simulink model "M1DCS_2_rust"  (R2022b)
settings: Solver=FixedStepDiscrete  StartTime=0.0  StopTime=5  FixedStep=deltaT  RelTol=1e-3
InitFcn:
  | %
  | % Initialization callback function
  | %
  | 
  | try
  |    % fprintf('\n Simulink control model!\n');
  | 
  |    % Get Simulink model directory
  |    [filepath,name,ext] = fileparts(which(bdroot));
  | 
  |    if ~strcmp(filepath,pwd)
  |       fprintf('\n Changing current directory to \n %s \n',filepath);
  |       cd(filepath);
  |    end
  | 
  | catch
  |    warning('Running the InitFcn from puSimulate script');
  | end
values from neighbouring files (symbols this model uses):
  CS_Kbal = [0.000534994973474 0.00340191071412 -9.47788829769e-05 0.00343343348513 -0.000647828526781 -0.000556821142243 -0.000534821819969 -0.00340176071448 9.48233962239e-05 -0.00343325428788 0.000647837590074 0.000556848416436 ... (1836 elements, 306x6)]    [SupportActuatorArrayConfig.mat]
  CS_ofl_SSdtC = ofl_SSdtC    [load_M1DCS_data.m]
  H_p_cyl_DT = c2d(H_p_cyl, T_ofl, 'foh')    [load_M1DCS_data.m]
  HPdyn = c2d(feedback(tf([kpp_, kpi_],[1 0])*Hv_*Pp,1), T_ofl,'foh')    [load_M1DCS_data.m]
  m1_HPk = mean(HPstiffvec)    [load_M1DCS_data.m]
  M_HP_OA = M_HP_OA + (1/6)*M_HP_seg{i_}    [load_M1DCS_data.m]
  OA_Kbal = [0.0131193522784 0 0.000573456323239 0.0120863820226 0 -0.000305081290389 0.0117152923831 0 0.000463979607413 0.0115338103781 0 -0.00185896787401 ... (2010 elements, 335x6)]    [SupportActuatorArrayConfig.mat]
  OA_ofl_SSdtC = ofl_SSdtC    [load_M1DCS_data.m]
  T_ofl = 0.01    [load_M1DCS_data.m]
undefined symbols (not defined in the file or in its folder): m1sys, M_HP_CS, S1_M1RBM2HP, S2_M1RBM2HP, S3_M1RBM2HP, S4_M1RBM2HP, S5_M1RBM2HP, S6_M1RBM2HP, S7_M1RBM2HP
libraries: ims_block_library x2
settings Model: SimulationMode=accelerator  Creator=RRomano  LastModifiedBy=rromano
settings SolverCC: AlgebraicLoopSolver=TrustRegion
settings DataIOCC: SaveOutput=off  SignalLogging=off  DSMLogging=off  SaveTime=off  ReturnWorkspaceOutputs=off
settings OptimizationCC: DefaultParameterBehavior=Inlined  GainParamInheritBuiltInType=on  UseFloatMulNetSlope=on  UseSpecifiedMinMax=on  InlineInvariantSignals=on  StrengthReduction=on  PassReuseOutputArgsAs=Individual arguments  ZeroExternalMemoryAtStartup=off  ZeroInternalMemoryAtStartup=off  NoFixptDivByZeroProtection=on  EfficientFloat2IntCast=on  LifeSpan=1000  SimCompilerOptimization=on  AccelVerboseBuild=on  OptimizeBlockOrder=speed  OptimizationPriority=Speed  OptimizationCustomize=off  MultiThreadedLoops=on  EfficientTunableParamExpr=on
settings DebuggingCC: InheritedTsInSrcMsg=none  MultiTaskRateTransMsg=warning  ParameterTunabilityLossMsg=error  UnconnectedInputMsg=warning  UnconnectedOutputMsg=warning  UnconnectedLineMsg=warning  SFUnexpectedBacktrackingDiag=warning  SFNoUnconditionalDefaultTransitionDiag=warning  SFExecutionAtInitializationDiag=none  SFMachineParentedDataDiag=warning  ArithmeticOperatorsInVariantConditions=warning
settings HardwareCC: ProdBitPerLong=64  ProdLongLongMode=on  ProdHWDeviceType=Intel->x86-64 (Linux 64)  TargetBitPerLong=64  TargetBitPerPointer=64  TargetBitPerSizeT=64  TargetBitPerPtrDiffT=64  TargetLongLongMode=on  TargetIntDivRoundTo=Zero  TargetEndianess=LittleEndian  TargetWordSize=64  TargetHWDeviceType=MATLAB Host  ProdEqTarget=off
settings ModelReferenceCC: EnableRefExpFcnMdlSchedulingChecks=on
settings SFSimCC: SimUseLocalCustomCode=off  MATLABDynamicMemAlloc=off  CustomCodeUndefinedFunction=UseInterfaceOnly
settings RTWCC: Description=Embedded Coder  SystemTargetFile=ert.tlc  GenCodeOnly=on  GenerateMakefile=off  TemplateMakefile=ert_default_tmf  GenerateReport=on  BuildConfiguration=Faster Runs  RTWCompilerOptimization=on  CheckMdlBeforeBuild=Warning  DLArmComputeVersion=19.05
settings CodeAppCC: ForceParamTrailComments=on  IgnoreCustomStorageClasses=off  OperatorAnnotations=on  SimulinkDataObjDesc=on  SFDataObjDesc=on  InsertBlockDesc=on
settings ERTTargetCC: TargetLangStandard=C99 (ISO)  GenerateSampleERTMain=on  CombineSignalStateStructs=on  SuppressErrorStatus=on  CodeInterfacePackaging=Reusable function  SupportNonFinite=off  SupportComplex=off  InlinedParameterPlacement=NonHierarchical  RootIOFormat=Structure reference  ERTCustomFileTemplate=example_file_process.tlc
settings ConfigComp: CovMetricSettings=dw  CovSaveCumulativeToWorkspaceVar=on  CovSaveSingleToWorkspaceVar=on  CovExternalEMLEnable=off

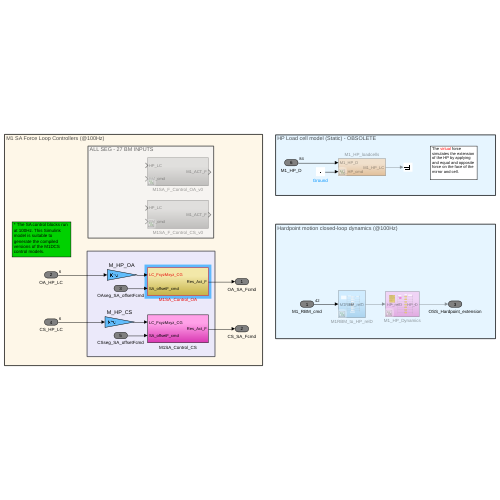
[thumbnail: Simulink's stored preview of the top-level diagram]
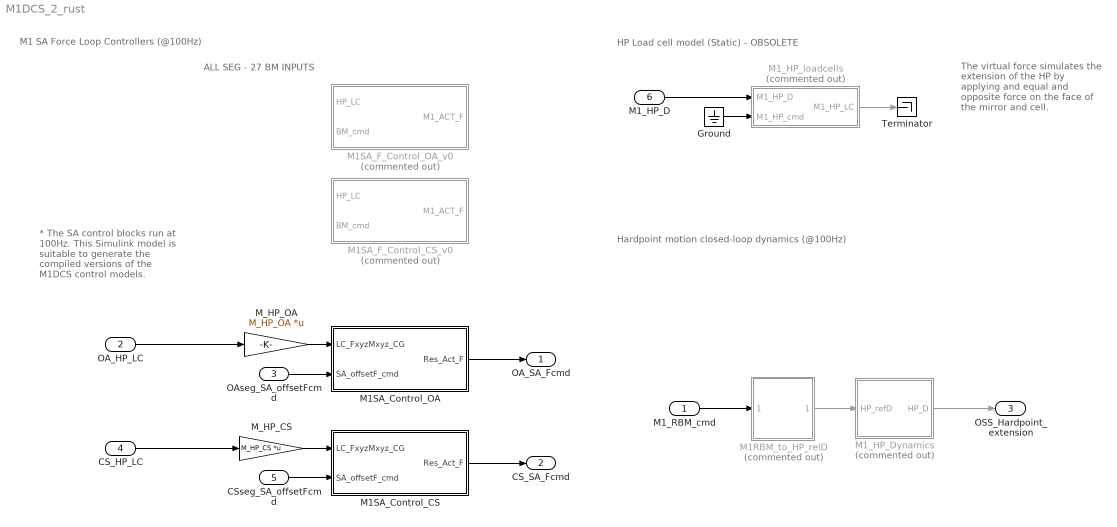
== system M1DCS_2_rust ==
  note: HP Load cell model (Static) - OBSOLETE
  note: Hardpoint motion closed-loop dynamics (@100Hz)
  note: ALL SEG - 27 BM INPUTS
  note: * The SA control blocks run at 100Hz. This Simulink model is suitable to generate the compiled versions of the M1DCS control models.
  note: M1 SA Force Loop Controllers (@100Hz)
  note: The virtual force simulates the extension of the HP by applying and equal and opposite force on the face of the mirror and cell.
  M1_RBM_cmd : Inport  PortDimensions=42
  OA_HP_LC : Inport  Port=2  PortDimensions=size(M_HP_OA,2)  SampleTime=T_ofl
  OAseg_SA_offsetFcmd : Inport  Port=3  SampleTime=T_ofl
  CS_HP_LC : Inport  Port=4  PortDimensions=size(M_HP_CS,2)  SampleTime=T_ofl
  CSseg_SA_offsetFcmd : Inport  Port=5  SampleTime=T_ofl
  M1_HP_D : Inport  Port=6  PortDimensions=84
  Ground : Ground
  M1RBM_to_HP_relD : Subsystem  Commented=on
  M1SA_Control_CS : Subsystem
  M1SA_Control_OA : Subsystem
  M1SA_F_Control_CS_v0 : Subsystem  Commented=on
  M1SA_F_Control_OA_v0 : Subsystem  Commented=on
  M1_HP_Dynamics : Subsystem  Commented=on
  M1_HP_loadcells : Subsystem  Commented=on
  M_HP_CS : Gain  Gain=M_HP_CS  Multiplication=Matrix(K*u)
  M_HP_OA : Gain  Gain=M_HP_OA  Multiplication=Matrix(K*u)
  Terminator : Terminator
  OA_SA_Fcmd : Outport  SampleTime=T_ofl  VectorParamsAs1DForOutWhenUnconnected=off
  CS_SA_Fcmd : Outport  Port=2  SampleTime=T_ofl  VectorParamsAs1DForOutWhenUnconnected=off
  OSS_Hardpoint_extension : Outport  Port=3  VectorParamsAs1DForOutWhenUnconnected=off
  wires:
  M1_RBM_cmd/1 -> M1RBM_to_HP_relD/1(M1RBM)
  M1SA_Control_CS/1(Res_Act_F) -> CS_SA_Fcmd/1
  CSseg_SA_offsetFcmd/1 -> M1SA_Control_CS/2(SA_offsetF_cmd)
  CS_HP_LC/1 -> M_HP_CS/1
  M1SA_Control_OA/1(Res_Act_F) -> OA_SA_Fcmd/1
  OA_HP_LC/1 -> M_HP_OA/1
  OAseg_SA_offsetFcmd/1 -> M1SA_Control_OA/2(SA_offsetF_cmd)
  M_HP_OA/1 -> M1SA_Control_OA/1(LC_FxyzMxyz_CG)
  M_HP_CS/1 -> M1SA_Control_CS/1(LC_FxyzMxyz_CG)
  M1_HP_Dynamics/1(HP_D) -> OSS_Hardpoint_extension/1
  M1RBM_to_HP_relD/1(HP_relD) -> M1_HP_Dynamics/1(HP_refD)
  M1_HP_loadcells/1(M1_HP_LC) -> Terminator/1
  M1_HP_D/1 -> M1_HP_loadcells/1(M1_HP_D)
  Ground/1 -> M1_HP_loadcells/2(M1_HP_cmd)

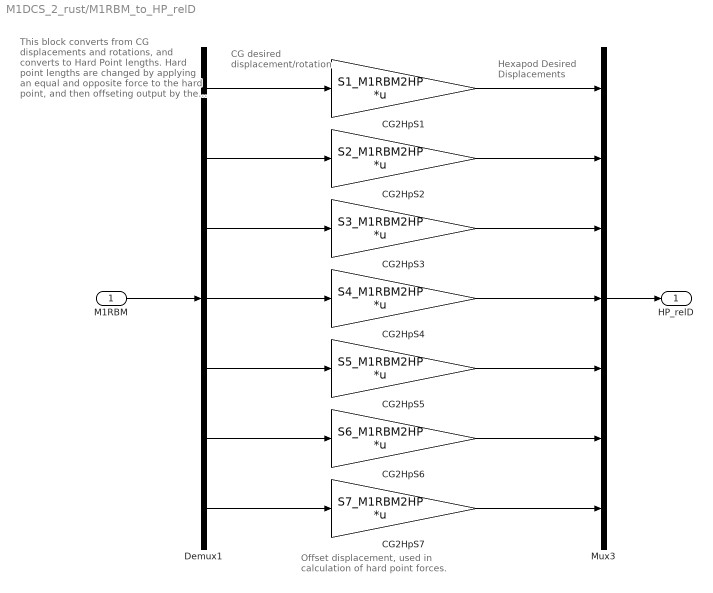
== system M1DCS_2_rust/M1RBM_to_HP_relD ==
  note: CG desired
      | displacement/rotation
  note: This block converts from CG displacements and rotations,
      | and converts to Hard Point lengths.  Hard point lengths are
      | changed by applying an equal and opposite force to the hard
      | point, and then offseting output by the commanded change
      | in position.
  note: Hexapod Desired
      | Displacements
  note: Offset displacement, used in calculation of hard point forces.
  M1RBM : Inport
  CG2HpS1 : Gain  Gain=S1_M1RBM2HP  Multiplication=Matrix(K*u)
  CG2HpS2 : Gain  Gain=S2_M1RBM2HP  Multiplication=Matrix(K*u)
  CG2HpS3 : Gain  Gain=S3_M1RBM2HP  Multiplication=Matrix(K*u)
  CG2HpS4 : Gain  Gain=S4_M1RBM2HP  Multiplication=Matrix(K*u)
  CG2HpS5 : Gain  Gain=S5_M1RBM2HP  Multiplication=Matrix(K*u)
  CG2HpS6 : Gain  Gain=S6_M1RBM2HP  Multiplication=Matrix(K*u)
  CG2HpS7 : Gain  Gain=S7_M1RBM2HP  Multiplication=Matrix(K*u)
  Demux1 : Demux  Outputs=6*ones(7,1)
  Mux3 : Mux  Inputs=6*ones(7,1)
  HP_relD : Outport  VectorParamsAs1DForOutWhenUnconnected=off
  wires:
  Mux3/1 -> HP_relD/1
  Demux1/2 -> CG2HpS2/1
  Demux1/3 -> CG2HpS3/1
  Demux1/4 -> CG2HpS4/1
  Demux1/5 -> CG2HpS5/1
  Demux1/6 -> CG2HpS6/1
  Demux1/1 -> CG2HpS1/1
  Demux1/7 -> CG2HpS7/1
  CG2HpS1/1 -> Mux3/1
  M1RBM/1 -> Demux1/1
  CG2HpS2/1 -> Mux3/2
  CG2HpS3/1 -> Mux3/3
  CG2HpS4/1 -> Mux3/4
  CG2HpS5/1 -> Mux3/5
  CG2HpS6/1 -> Mux3/6
  CG2HpS7/1 -> Mux3/7

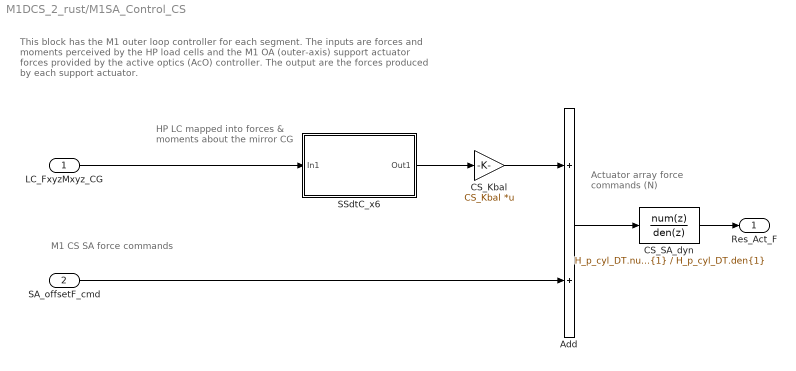
== system M1DCS_2_rust/M1SA_Control_CS ==
  note: This block has the M1 outer loop controller for each segment. The inputs are forces and moments perceived by the HP load cells and the M1 OA (outer-axis) support actuator forces provided by the active optics (AcO) controller. The output are the forces produced by each support actuator.
  note: Actuator array
      | force commands (N)
  note: M1 CS SA
      | force commands
  note: HP LC mapped into forces & moments about the mirror CG
  LC_FxyzMxyz_CG : Inport  PortDimensions=size(M_HP_CS,1)  SampleTime=T_ofl
  SA_offsetF_cmd : Inport  Port=2  PortDimensions=size(CS_Kbal,1)  SampleTime=T_ofl
  Add : Sum
  CS_Kbal : Gain  Gain=CS_Kbal  Multiplication=Matrix(K*u)
  CS_SA_dyn : DiscreteTransferFcn  Numerator=H_p_cyl_DT.num{1}  Denominator=H_p_cyl_DT.den{1}  SampleTime=T_ofl  a0EqualsOne=on
  SSdtC_x6 : Subsystem
  Res_Act_F : Outport  VectorParamsAs1DForOutWhenUnconnected=off
  wires:
  Add/1 -> CS_SA_dyn/1
  SA_offsetF_cmd/1 -> Add/2
  LC_FxyzMxyz_CG/1 -> SSdtC_x6/1(In1)
  SSdtC_x6/1(Out1) -> CS_Kbal/1
  CS_Kbal/1 -> Add/1
  CS_SA_dyn/1 -> Res_Act_F/1

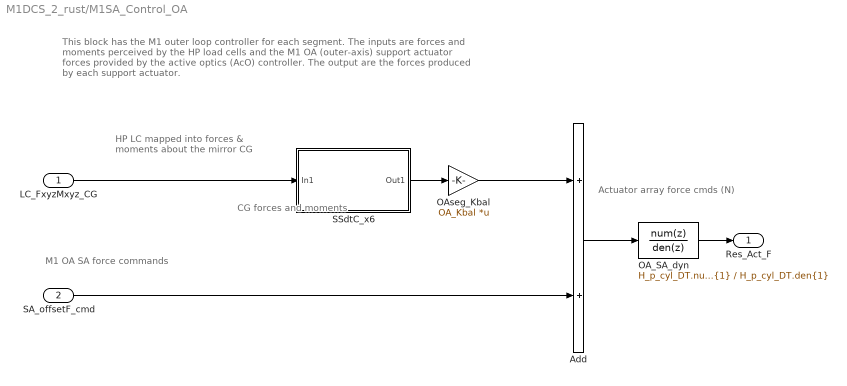
== system M1DCS_2_rust/M1SA_Control_OA ==
  note: M1 OA SA force
      | commands
  note: This block has the M1 outer loop controller for each segment. The inputs are forces and moments perceived by the HP load cells and the M1 OA (outer-axis) support actuator forces provided by the active optics (AcO) controller. The output are the forces produced by each support actuator.
  note: CG forces
      | and moments
  note: Actuator array
      | force cmds (N)
  note: HP LC mapped into forces & moments about the mirror CG
  LC_FxyzMxyz_CG : Inport  PortDimensions=size(M_HP_OA,1)  SampleTime=T_ofl
  SA_offsetF_cmd : Inport  Port=2  PortDimensions=size(OA_Kbal,1)  SampleTime=T_ofl
  Add : Sum
  OA_SA_dyn : DiscreteTransferFcn  Numerator=H_p_cyl_DT.num{1}  Denominator=H_p_cyl_DT.den{1}  SampleTime=T_ofl  a0EqualsOne=on
  OAseg_Kbal : Gain  Gain=OA_Kbal  Multiplication=Matrix(K*u)
  SSdtC_x6 : Subsystem
  Res_Act_F : Outport  VectorParamsAs1DForOutWhenUnconnected=off
  wires:
  SA_offsetF_cmd/1 -> Add/2
  OAseg_Kbal/1 -> Add/1
  LC_FxyzMxyz_CG/1 -> SSdtC_x6/1(In1)
  SSdtC_x6/1(Out1) -> OAseg_Kbal/1
  OA_SA_dyn/1 -> Res_Act_F/1
  Add/1 -> OA_SA_dyn/1

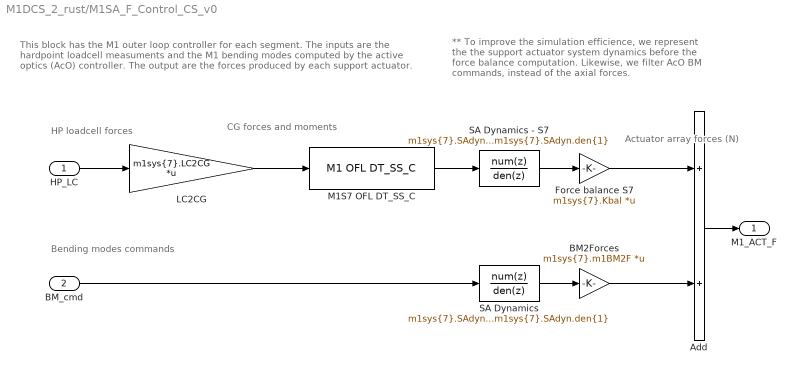
== system M1DCS_2_rust/M1SA_F_Control_CS_v0 ==
  note: This block has the M1 outer loop controller for each segment. The inputs are the hardpoint loadcell measuments and the M1 bending modes computed by the active optics (AcO) controller. The output are the forces produced by each support actuator.
  note: Actuator array
      | forces (N)
  note: HP loadcell
      | forces
  note: ** To improve the simulation efficience, we represent the the support actuator system dynamics before the force balance computation. Likewise, we filter AcO BM commands, instead of the axial forces.
  note: Bending modes
      | commands
  note: CG forces
      | and moments
  HP_LC : Inport  PortDimensions=size(m1sys{7}.LC2CG,1)  SampleTime=m1sys{7}.ofl.SSdtC{1}.Ts
  BM_cmd : Inport  Port=2  PortDimensions=n_bm  SampleTime=m1sys{7}.ofl.SSdtC{1}.Ts
  Add : Sum
  BM2Forces : Gain  Gain=m1sys{7}.m1BM2F  Multiplication=Matrix(K*u)
  Force balance S7 : Gain  Gain=m1sys{7}.Kbal  Multiplication=Matrix(K*u)
  LC2CG : Gain  Gain=m1sys{7}.LC2CG  Multiplication=Matrix(K*u)
  M1S7 OFL DT_SS_C : ims_block_library/M1 OFL DT_SS_C  dt_SS_struct=m1sys{7}.ofl.SSdtC
  SA Dynamics : DiscreteTransferFcn  Numerator=m1sys{7}.SAdyn.num{1}  Denominator=m1sys{7}.SAdyn.den{1}  SampleTime=m1sys{7}.ofl.SSdtC{1}.Ts  a0EqualsOne=on
  SA Dynamics - S7 : DiscreteTransferFcn  Numerator=m1sys{7}.SAdyn.num{1}  Denominator=m1sys{7}.SAdyn.den{1}  SampleTime=m1sys{7}.ofl.SSdtC{1}.Ts  a0EqualsOne=on
  M1_ACT_F : Outport  VectorParamsAs1DForOutWhenUnconnected=off
  wires:
  Force balance S7/1 -> Add/1
  Add/1 -> M1_ACT_F/1
  HP_LC/1 -> LC2CG/1
  SA Dynamics - S7/1 -> Force balance S7/1
  BM2Forces/1 -> Add/2
  M1S7 OFL DT_SS_C/1 -> SA Dynamics - S7/1
  LC2CG/1 -> M1S7 OFL DT_SS_C/1
  BM_cmd/1 -> SA Dynamics/1
  SA Dynamics/1 -> BM2Forces/1

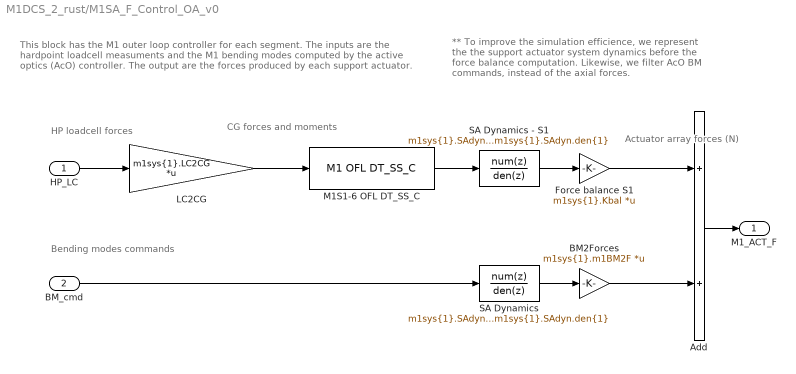
== system M1DCS_2_rust/M1SA_F_Control_OA_v0 ==
  note: ** To improve the simulation efficience, we represent the the support actuator system dynamics before the force balance computation. Likewise, we filter AcO BM commands, instead of the axial forces.
  note: Bending modes
      | commands
  note: This block has the M1 outer loop controller for each segment. The inputs are the hardpoint loadcell measuments and the M1 bending modes computed by the active optics (AcO) controller. The output are the forces produced by each support actuator.
  note: CG forces
      | and moments
  note: Actuator array
      | forces (N)
  note: HP loadcell
      | forces
  HP_LC : Inport  PortDimensions=size(m1sys{1}.LC2CG,1)  SampleTime=m1sys{1}.ofl.SSdtC{1}.Ts
  BM_cmd : Inport  Port=2  PortDimensions=n_bm  SampleTime=m1sys{1}.ofl.SSdtC{1}.Ts
  Add : Sum
  BM2Forces : Gain  Gain=m1sys{1}.m1BM2F  Multiplication=Matrix(K*u)
  Force balance S1 : Gain  Gain=m1sys{1}.Kbal  Multiplication=Matrix(K*u)
  LC2CG : Gain  Gain=m1sys{1}.LC2CG  Multiplication=Matrix(K*u)
  M1S1-6 OFL DT_SS_C : ims_block_library/M1 OFL DT_SS_C  dt_SS_struct=m1sys{1}.ofl.SSdtC
  SA Dynamics : DiscreteTransferFcn  Numerator=m1sys{1}.SAdyn.num{1}  Denominator=m1sys{1}.SAdyn.den{1}  SampleTime=m1sys{1}.ofl.SSdtC{1}.Ts  a0EqualsOne=on
  SA Dynamics - S1 : DiscreteTransferFcn  Numerator=m1sys{1}.SAdyn.num{1}  Denominator=m1sys{1}.SAdyn.den{1}  SampleTime=m1sys{1}.ofl.SSdtC{1}.Ts  a0EqualsOne=on
  M1_ACT_F : Outport  VectorParamsAs1DForOutWhenUnconnected=off
  wires:
  Force balance S1/1 -> Add/1
  M1S1-6 OFL DT_SS_C/1 -> SA Dynamics - S1/1
  HP_LC/1 -> LC2CG/1
  SA Dynamics - S1/1 -> Force balance S1/1
  BM_cmd/1 -> SA Dynamics/1
  LC2CG/1 -> M1S1-6 OFL DT_SS_C/1
  Add/1 -> M1_ACT_F/1
  SA Dynamics/1 -> BM2Forces/1
  BM2Forces/1 -> Add/2

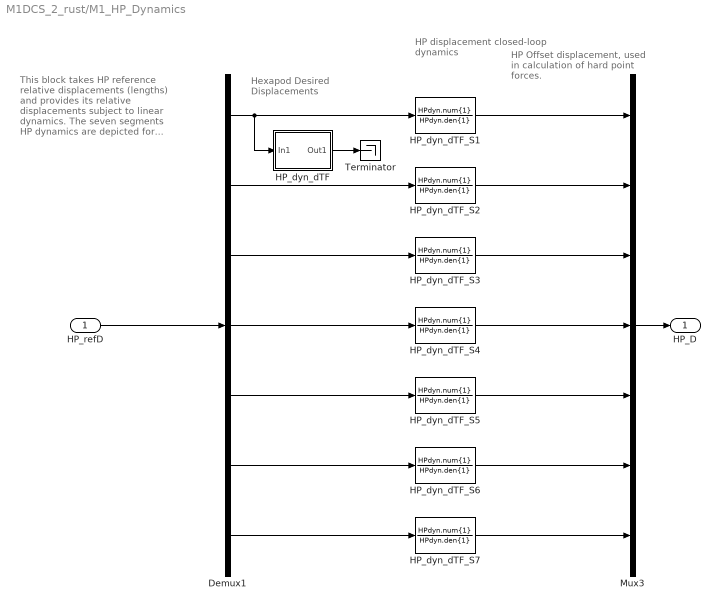
== system M1DCS_2_rust/M1_HP_Dynamics ==
  note: This block takes HP reference relative displacements (lengths) and provides its relative displacements subject to linear dynamics. The seven segments HP dynamics are depicted for illustration. One is supposed to build the single segmen dynamcs ( magenta block HP_dyn_dTF ). Then, the code is cloned for the multiple segments.
  note: Hexapod Desired
      | Displacements
  note: HP Offset displacement, used in calculation of hard point forces.
  note: HP displacement closed-loop dynamics
  HP_refD : Inport
  Demux1 : Demux  Outputs=6*ones(7,1)
  HP_dyn_dTF : Subsystem
  HP_dyn_dTF_S{1..7} (7 alike) : DiscreteTransferFcn  Numerator=HPdyn.num{1}  Denominator=HPdyn.den{1}  SampleTime=HPdyn.Ts  a0EqualsOne=on
  Mux3 : Mux  Inputs=6*ones(7,1)
  Terminator : Terminator
  HP_D : Outport  VectorParamsAs1DForOutWhenUnconnected=off
  wires:
  Mux3/1 -> HP_D/1
  Demux1/1 -> HP_dyn_dTF/1(In1), HP_dyn_dTF_S1/1
  HP_refD/1 -> Demux1/1
  Demux1/2 -> HP_dyn_dTF_S2/1
  Demux1/3 -> HP_dyn_dTF_S3/1
  Demux1/4 -> HP_dyn_dTF_S4/1
  Demux1/5 -> HP_dyn_dTF_S5/1
  Demux1/6 -> HP_dyn_dTF_S6/1
  Demux1/7 -> HP_dyn_dTF_S7/1
  HP_dyn_dTF_S1/1 -> Mux3/1
  HP_dyn_dTF_S2/1 -> Mux3/2
  HP_dyn_dTF_S3/1 -> Mux3/3
  HP_dyn_dTF_S4/1 -> Mux3/4
  HP_dyn_dTF_S5/1 -> Mux3/5
  HP_dyn_dTF_S6/1 -> Mux3/6
  HP_dyn_dTF_S7/1 -> Mux3/7
  HP_dyn_dTF/1(Out1) -> Terminator/1

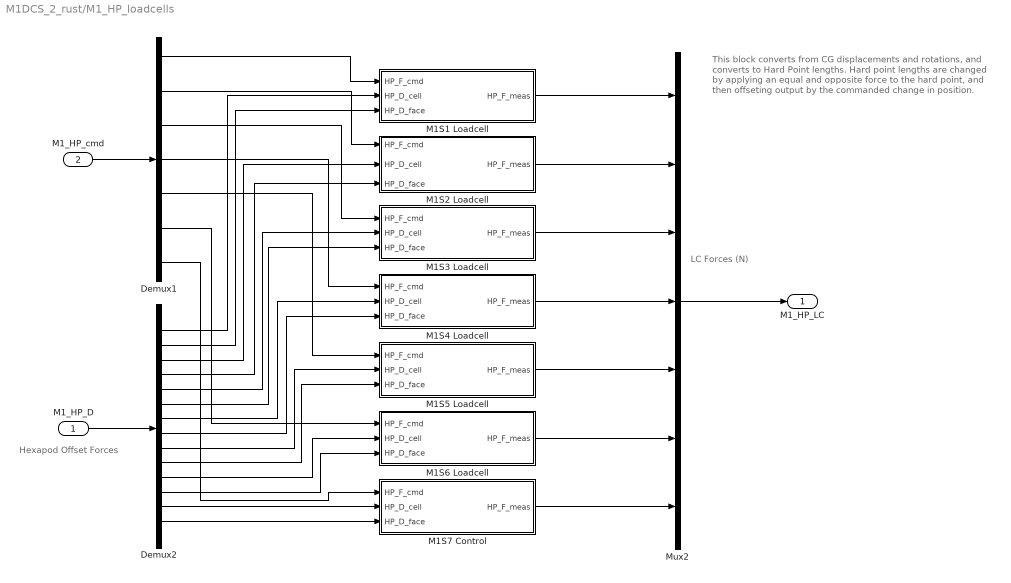
== system M1DCS_2_rust/M1_HP_loadcells ==
  note: This block converts from CG displacements and rotations,
      | and converts to Hard Point lengths.  Hard point lengths are
      | changed by applying an equal and opposite force to the hard
      | point, and then offseting output by the commanded change
      | in position.
  note: Hexapod Offset Forces
  note: LC Forces (N)
  M1_HP_D : Inport
  M1_HP_cmd : Inport  Port=2
  Demux1 : Demux  Outputs=6*ones(7,1)
  Demux2 : Demux  Outputs=6*ones(14,1);%6*ones(7,1)
  M1S1 Loadcell : Subsystem
  M1S2 Loadcell : Subsystem
  M1S3 Loadcell : Subsystem
  M1S4 Loadcell : Subsystem
  M1S5 Loadcell : Subsystem
  M1S6 Loadcell : Subsystem
  M1S7 Control : Subsystem
  Mux2 : Mux  Inputs=7
  M1_HP_LC : Outport  VectorParamsAs1DForOutWhenUnconnected=off
  wires:
  Demux2/9 -> M1S5 Loadcell/2(HP_D_cell)
  Demux2/3 -> M1S2 Loadcell/2(HP_D_cell)
  Demux2/5 -> M1S3 Loadcell/2(HP_D_cell)
  Demux2/13 -> M1S7 Control/2(HP_D_cell)
  Demux2/11 -> M1S6 Loadcell/2(HP_D_cell)
  Demux2/4 -> M1S2 Loadcell/3(HP_D_face)
  Demux2/6 -> M1S3 Loadcell/3(HP_D_face)
  Demux2/10 -> M1S5 Loadcell/3(HP_D_face)
  Demux2/12 -> M1S6 Loadcell/3(HP_D_face)
  Demux2/14 -> M1S7 Control/3(HP_D_face)
  M1_HP_D/1 -> Demux2/1
  M1S1 Loadcell/1(HP_F_meas) -> Mux2/1
  M1S2 Loadcell/1(HP_F_meas) -> Mux2/2
  M1S3 Loadcell/1(HP_F_meas) -> Mux2/3
  M1S5 Loadcell/1(HP_F_meas) -> Mux2/5
  M1S6 Loadcell/1(HP_F_meas) -> Mux2/6
  M1S7 Control/1(HP_F_meas) -> Mux2/7
  Demux2/2 -> M1S1 Loadcell/3(HP_D_face)
  Demux2/1 -> M1S1 Loadcell/2(HP_D_cell)
  M1S4 Loadcell/1(HP_F_meas) -> Mux2/4
  Demux2/7 -> M1S4 Loadcell/2(HP_D_cell)
  Demux2/8 -> M1S4 Loadcell/3(HP_D_face)
  M1_HP_cmd/1 -> Demux1/1
  Demux1/1 -> M1S1 Loadcell/1(HP_F_cmd)
  Demux1/2 -> M1S2 Loadcell/1(HP_F_cmd)
  Demux1/3 -> M1S3 Loadcell/1(HP_F_cmd)
  Demux1/4 -> M1S4 Loadcell/1(HP_F_cmd)
  Demux1/5 -> M1S5 Loadcell/1(HP_F_cmd)
  Demux1/6 -> M1S6 Loadcell/1(HP_F_cmd)
  Demux1/7 -> M1S7 Control/1(HP_F_cmd)
  Mux2/1 -> M1_HP_LC/1

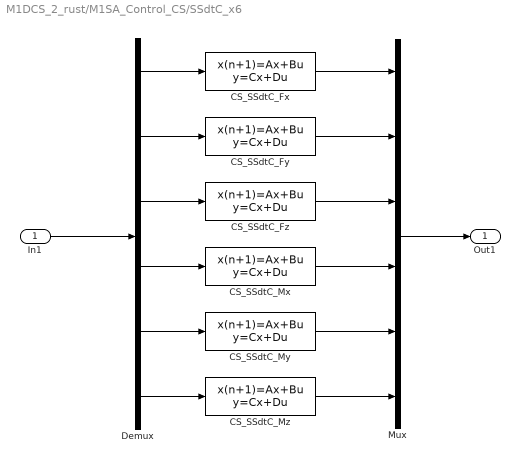
== system M1DCS_2_rust/M1SA_Control_CS/SSdtC_x6 ==
  In1 : Inport
  CS_SSdtC_Fx : DiscreteStateSpace  A=CS_ofl_SSdtC.A  B=CS_ofl_SSdtC.B  C=CS_ofl_SSdtC.C  D=CS_ofl_SSdtC.D  SampleTime=CS_ofl_SSdtC.Ts
  CS_SSdtC_Fy : DiscreteStateSpace  A=CS_ofl_SSdtC.A  B=CS_ofl_SSdtC.B  C=CS_ofl_SSdtC.C  D=CS_ofl_SSdtC.D  SampleTime=CS_ofl_SSdtC.Ts
  CS_SSdtC_Fz : DiscreteStateSpace  A=CS_ofl_SSdtC.A  B=CS_ofl_SSdtC.B  C=CS_ofl_SSdtC.C  D=CS_ofl_SSdtC.D  SampleTime=CS_ofl_SSdtC.Ts
  CS_SSdtC_Mx : DiscreteStateSpace  A=CS_ofl_SSdtC.A  B=CS_ofl_SSdtC.B  C=CS_ofl_SSdtC.C  D=CS_ofl_SSdtC.D  SampleTime=CS_ofl_SSdtC.Ts
  CS_SSdtC_My : DiscreteStateSpace  A=CS_ofl_SSdtC.A  B=CS_ofl_SSdtC.B  C=CS_ofl_SSdtC.C  D=CS_ofl_SSdtC.D  SampleTime=CS_ofl_SSdtC.Ts
  CS_SSdtC_Mz : DiscreteStateSpace  A=CS_ofl_SSdtC.A  B=CS_ofl_SSdtC.B  C=CS_ofl_SSdtC.C  D=CS_ofl_SSdtC.D  SampleTime=CS_ofl_SSdtC.Ts
  Demux : Demux  Outputs=6
  Mux : Mux  Inputs=6
  Out1 : Outport
  wires:
  In1/1 -> Demux/1
  Demux/1 -> CS_SSdtC_Fx/1
  CS_SSdtC_Fx/1 -> Mux/1
  Mux/1 -> Out1/1
  Demux/2 -> CS_SSdtC_Fy/1
  CS_SSdtC_Fy/1 -> Mux/2
  Demux/3 -> CS_SSdtC_Fz/1
  CS_SSdtC_Fz/1 -> Mux/3
  Demux/4 -> CS_SSdtC_Mx/1
  CS_SSdtC_Mx/1 -> Mux/4
  Demux/5 -> CS_SSdtC_My/1
  CS_SSdtC_My/1 -> Mux/5
  Demux/6 -> CS_SSdtC_Mz/1
  CS_SSdtC_Mz/1 -> Mux/6

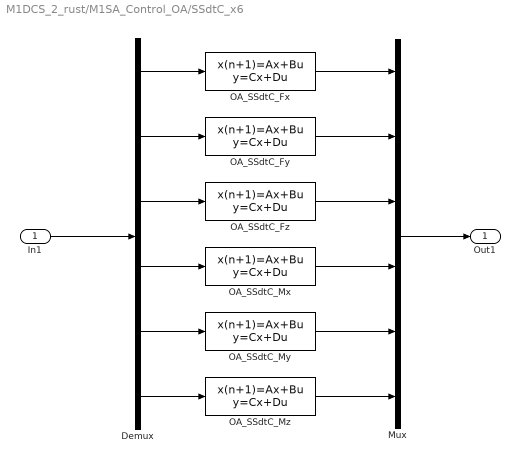
== system M1DCS_2_rust/M1SA_Control_OA/SSdtC_x6 ==
  In1 : Inport
  Demux : Demux  Outputs=6
  Mux : Mux  Inputs=6
  OA_SSdtC_Fx : DiscreteStateSpace  A=OA_ofl_SSdtC.A  B=OA_ofl_SSdtC.B  C=OA_ofl_SSdtC.C  D=OA_ofl_SSdtC.D  SampleTime=OA_ofl_SSdtC.Ts
  OA_SSdtC_Fy : DiscreteStateSpace  A=OA_ofl_SSdtC.A  B=OA_ofl_SSdtC.B  C=OA_ofl_SSdtC.C  D=OA_ofl_SSdtC.D  SampleTime=OA_ofl_SSdtC.Ts
  OA_SSdtC_Fz : DiscreteStateSpace  A=OA_ofl_SSdtC.A  B=OA_ofl_SSdtC.B  C=OA_ofl_SSdtC.C  D=OA_ofl_SSdtC.D  SampleTime=OA_ofl_SSdtC.Ts
  OA_SSdtC_Mx : DiscreteStateSpace  A=OA_ofl_SSdtC.A  B=OA_ofl_SSdtC.B  C=OA_ofl_SSdtC.C  D=OA_ofl_SSdtC.D  SampleTime=OA_ofl_SSdtC.Ts
  OA_SSdtC_My : DiscreteStateSpace  A=OA_ofl_SSdtC.A  B=OA_ofl_SSdtC.B  C=OA_ofl_SSdtC.C  D=OA_ofl_SSdtC.D  SampleTime=OA_ofl_SSdtC.Ts
  OA_SSdtC_Mz : DiscreteStateSpace  A=OA_ofl_SSdtC.A  B=OA_ofl_SSdtC.B  C=OA_ofl_SSdtC.C  D=OA_ofl_SSdtC.D  SampleTime=OA_ofl_SSdtC.Ts
  Out1 : Outport
  wires:
  In1/1 -> Demux/1
  Demux/1 -> OA_SSdtC_Fx/1
  OA_SSdtC_Fx/1 -> Mux/1
  Mux/1 -> Out1/1
  Demux/2 -> OA_SSdtC_Fy/1
  Demux/3 -> OA_SSdtC_Fz/1
  Demux/4 -> OA_SSdtC_Mx/1
  Demux/5 -> OA_SSdtC_My/1
  Demux/6 -> OA_SSdtC_Mz/1
  OA_SSdtC_Fy/1 -> Mux/2
  OA_SSdtC_Fz/1 -> Mux/3
  OA_SSdtC_Mx/1 -> Mux/4
  OA_SSdtC_My/1 -> Mux/5
  OA_SSdtC_Mz/1 -> Mux/6

== system M1DCS_2_rust/M1_HP_Dynamics/HP_dyn_dTF ==
  In1 : Inport
  HP_dyn_dTF : DiscreteTransferFcn  Numerator=HPdyn.num{1}  Denominator=HPdyn.den{1}  SampleTime=HPdyn.Ts  a0EqualsOne=on
  Out1 : Outport
  wires:
  HP_dyn_dTF/1 -> Out1/1
  In1/1 -> HP_dyn_dTF/1

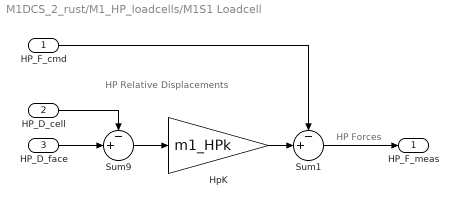
== system M1DCS_2_rust/M1_HP_loadcells/M1S1 Loadcell ==
  note: HP Forces
  note: HP Relative
      | Displacements
  HP_F_cmd : Inport
  HP_D_cell : Inport  Port=2
  HP_D_face : Inport  Port=3
  HpK : Gain  Gain=m1_HPk
  Sum1 : Sum  Inputs=-+|
  Sum9 : Sum  Inputs=-+|
  HP_F_meas : Outport  VectorParamsAs1DForOutWhenUnconnected=off
  wires:
  HP_D_cell/1 -> Sum9/1
  HP_D_face/1 -> Sum9/2
  Sum9/1 -> HpK/1
  HpK/1 -> Sum1/2
  Sum1/1 -> HP_F_meas/1
  HP_F_cmd/1 -> Sum1/1

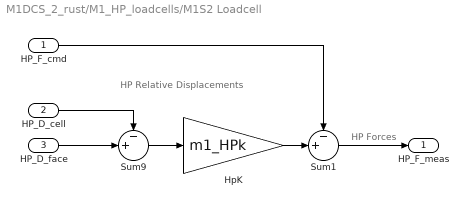
== system M1DCS_2_rust/M1_HP_loadcells/M1S2 Loadcell ==
  note: HP Relative
      | Displacements
  note: HP Forces
  HP_F_cmd : Inport
  HP_D_cell : Inport  Port=2
  HP_D_face : Inport  Port=3
  HpK : Gain  Gain=m1_HPk
  Sum1 : Sum  Inputs=-+|
  Sum9 : Sum  Inputs=-+|
  HP_F_meas : Outport  VectorParamsAs1DForOutWhenUnconnected=off
  wires:
  HP_D_face/1 -> Sum9/2
  HP_D_cell/1 -> Sum9/1
  HP_F_cmd/1 -> Sum1/1
  HpK/1 -> Sum1/2
  Sum1/1 -> HP_F_meas/1
  Sum9/1 -> HpK/1

== system M1DCS_2_rust/M1_HP_loadcells/M1S3 Loadcell ==
  note: HP Relative
      | Displacements
  note: HP Forces
  HP_F_cmd : Inport
  HP_D_cell : Inport  Port=2
  HP_D_face : Inport  Port=3
  HpK : Gain  Gain=m1_HPk
  Sum1 : Sum  Inputs=-+|
  Sum9 : Sum  Inputs=-+|
  HP_F_meas : Outport  VectorParamsAs1DForOutWhenUnconnected=off
  wires:
  HP_D_face/1 -> Sum9/2
  HP_D_cell/1 -> Sum9/1
  HP_F_cmd/1 -> Sum1/1
  HpK/1 -> Sum1/2
  Sum1/1 -> HP_F_meas/1
  Sum9/1 -> HpK/1

== system M1DCS_2_rust/M1_HP_loadcells/M1S4 Loadcell ==
  note: HP Relative
      | Displacements
  note: HP Forces
  HP_F_cmd : Inport
  HP_D_cell : Inport  Port=2
  HP_D_face : Inport  Port=3
  HpK : Gain  Gain=m1_HPk
  Sum1 : Sum  Inputs=-+|
  Sum9 : Sum  Inputs=-+|
  HP_F_meas : Outport  VectorParamsAs1DForOutWhenUnconnected=off
  wires:
  HP_D_face/1 -> Sum9/2
  HP_D_cell/1 -> Sum9/1
  HP_F_cmd/1 -> Sum1/1
  HpK/1 -> Sum1/2
  Sum1/1 -> HP_F_meas/1
  Sum9/1 -> HpK/1

== system M1DCS_2_rust/M1_HP_loadcells/M1S5 Loadcell ==
  note: HP Relative
      | Displacements
  note: HP Forces
  HP_F_cmd : Inport
  HP_D_cell : Inport  Port=2
  HP_D_face : Inport  Port=3
  HpK : Gain  Gain=m1_HPk
  Sum1 : Sum  Inputs=-+|
  Sum9 : Sum  Inputs=-+|
  HP_F_meas : Outport  VectorParamsAs1DForOutWhenUnconnected=off
  wires:
  HP_D_face/1 -> Sum9/2
  HP_D_cell/1 -> Sum9/1
  HP_F_cmd/1 -> Sum1/1
  HpK/1 -> Sum1/2
  Sum1/1 -> HP_F_meas/1
  Sum9/1 -> HpK/1

== system M1DCS_2_rust/M1_HP_loadcells/M1S6 Loadcell ==
  note: HP Relative
      | Displacements
  note: HP Forces
  HP_F_cmd : Inport
  HP_D_cell : Inport  Port=2
  HP_D_face : Inport  Port=3
  HpK : Gain  Gain=m1_HPk
  Sum1 : Sum  Inputs=-+|
  Sum9 : Sum  Inputs=-+|
  HP_F_meas : Outport  VectorParamsAs1DForOutWhenUnconnected=off
  wires:
  HP_D_face/1 -> Sum9/2
  HP_D_cell/1 -> Sum9/1
  HP_F_cmd/1 -> Sum1/1
  HpK/1 -> Sum1/2
  Sum1/1 -> HP_F_meas/1
  Sum9/1 -> HpK/1

== system M1DCS_2_rust/M1_HP_loadcells/M1S7 Control ==
  note: HP Relative
      | Displacements
  note: HP Forces
  HP_F_cmd : Inport
  HP_D_cell : Inport  Port=2
  HP_D_face : Inport  Port=3
  HpK : Gain  Gain=m1_HPk
  Sum1 : Sum  Inputs=-+|
  Sum9 : Sum  Inputs=-+|
  HP_F_meas : Outport  VectorParamsAs1DForOutWhenUnconnected=off
  wires:
  HP_D_face/1 -> Sum9/2
  HP_D_cell/1 -> Sum9/1
  HP_F_cmd/1 -> Sum1/1
  HpK/1 -> Sum1/2
  Sum1/1 -> HP_F_meas/1
  Sum9/1 -> HpK/1
